simulink model "ksp_zad16"  (Simulink 2.20)
settings: Solver=ode45  StartTime=0.0  StopTime=90.0  RelTol=1e-3  AbsTol=1e-6
settings Model: ConsistencyChecking=off  RTWPlaceOutputsASAP=off

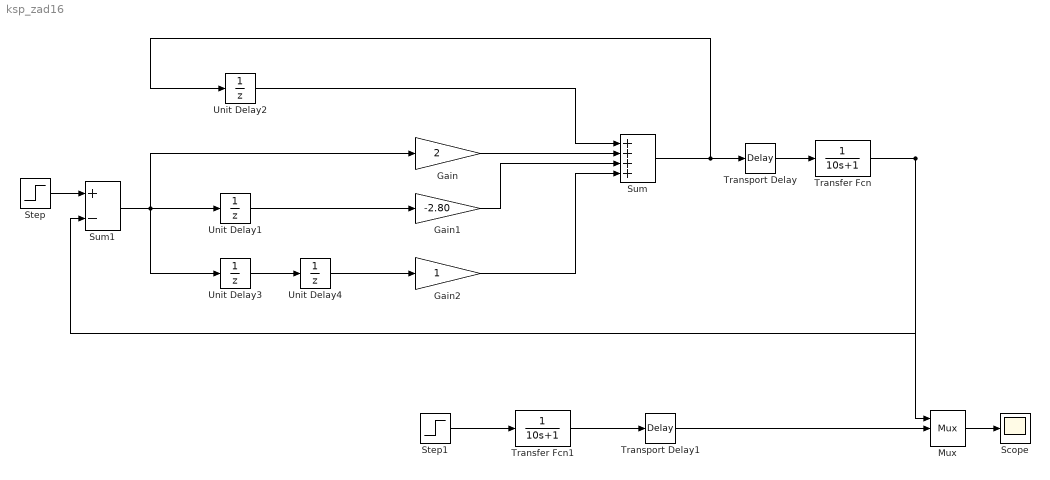
== system ksp_zad16 ==
  Gain : Gain  Gain=2
  Gain1 : Gain  Gain=-2.80
  Gain2 : Gain  Gain=1
  Mux : Mux  Inputs=3
  Scope : Scope
      settings: TickLabels=on  TimeRange=auto  YMin=-0.05  YMax=1.5  SaveToWorkspace=off  SaveName=ScopeData
  Step : Step  Time=1  Before=0  After=1
  Step1 : Step  Time=1  Before=0  After=1
  Sum : Sum  Inputs=++++
  Sum1 : Sum  Inputs=+-
  Transfer Fcn : TransferFcn  Numerator=[1]  Denominator=[10 1]
  Transfer Fcn1 : TransferFcn  Numerator=[1]  Denominator=[10 1]
  Transport Delay : TransportDelay  DelayTime=2  InitialInput=0  BufferSize=1024
  Transport Delay1 : TransportDelay  DelayTime=2  InitialInput=0  BufferSize=1024
  Unit Delay{1..4} (4 alike) : UnitDelay  X0=0  SampleTime=1
  wires:
  Step/1 -> Sum1/1
  Gain2/1 -> Sum/4
  Unit Delay2/1 -> Sum/1
  Gain1/1 -> Sum/3
  Gain/1 -> Sum/2
  Sum1/1 -> Gain/1, Unit Delay1/1, Unit Delay3/1
  Unit Delay4/1 -> Gain2/1
  Unit Delay3/1 -> Unit Delay4/1
  Unit Delay1/1 -> Gain1/1
  Sum/1 -> Unit Delay2/1, Transport Delay/1
  Mux/1 -> Scope/1
  Step1/1 -> Transfer Fcn1/1
  Transfer Fcn1/1 -> Transport Delay1/1
  Transport Delay1/1 -> Mux/2
  Transfer Fcn/1 -> Sum1/2, Mux/1
  Transport Delay/1 -> Transfer Fcn/1
